simulink model "chap04_CA1"  (R2021a)
settings: Solver=FixedStepDiscrete  StartTime=0.0  StopTime=30  FixedStep=0.001  RelTol=1e-3
undefined symbols (not defined in the file): DiscIntNeverNeededParam
libraries: simulink x4
(part 3 of 4)

== system chap04_CA1/Subsystem/Subsystem2/Subsystem6 ==
  xx2 : Inport
  xx1 : Inport  Port=2
  xx4 : Inport  Port=3
  xx6 : Inport  Port=4
  vx2 : Inport  Port=5
  vx1 : Inport  Port=6
  vx4 : Inport  Port=7
  vx6 : Inport  Port=8
  Add : Sum
  Add{1,4,6,8} (4 alike) : Sum  Inputs=-+
  Add2 : Sum  Inputs=+-
  Add5 : Sum  Inputs=+++
  Add7 : Sum  Inputs=+-
  Add9 : Sum  Inputs=+++
  Constant1 : Constant  Value=0.5
  Constant2 : Constant  Value=1.0
  Constant3 : Constant  Value=0.5
  Constant4 : Constant  Value=1.0
  Constant5 : Constant  Value=1.5
  Constant6 : Constant  Value=1.5
  Gain : Gain  Gain=-5
  Product{3..5,7..9} (6 alike) : Product
  p2x : Outport
  wires:
  Product4/1 -> Add5/2
  Product5/1 -> Add5/3
  Constant3/1 -> Product4/1
  Add4/1 -> Product4/2
  xx2/1 -> Add1/2, Add4/2, Add2/1
  Constant4/1 -> Product5/2
  Add2/1 -> Product5/1
  xx4/1 -> Add4/1
  xx1/1 -> Add2/2
  xx6/1 -> Add1/1
  Constant5/1 -> Product3/1
  Add1/1 -> Product3/2
  Product3/1 -> Add5/1
  Product7/1 -> Add9/1
  Add6/1 -> Product7/2
  Constant6/1 -> Product7/1
  vx6/1 -> Add6/1
  vx1/1 -> Add7/2
  vx4/1 -> Add8/1
  Add7/1 -> Product9/1
  Constant2/1 -> Product9/2
  vx2/1 -> Add7/1, Add8/2, Add6/2
  Add8/1 -> Product8/2
  Constant1/1 -> Product8/1
  Product9/1 -> Add9/3
  Product8/1 -> Add9/2
  Add5/1 -> Add/1
  Add/1 -> Gain/1
  Gain/1 -> p2x/1
  Add9/1 -> Add/2

== system chap04_CA1/Subsystem/Subsystem3/Subsystem1 ==
  xy4 : Inport
  xy2 : Inport  Port=2
  xy3 : Inport  Port=3
  xy5 : Inport  Port=4
  vy4 : Inport  Port=5
  vy2 : Inport  Port=6
  vy3 : Inport  Port=7
  vy5 : Inport  Port=8
  Add : Sum
  Add{1,4,6,8} (4 alike) : Sum  Inputs=-+
  Add2 : Sum  Inputs=+-
  Add5 : Sum  Inputs=+++
  Add7 : Sum  Inputs=+-
  Add9 : Sum  Inputs=+++
  Constant3 : Constant  Value=1.0
  Constant4 : Constant  Value=0.5
  Constant5 : Constant  Value=1.2
  Constant6 : Constant  Value=1.0
  Constant7 : Constant  Value=0.5
  Constant8 : Constant  Value=1.2
  Gain : Gain  Gain=-5.0
  Product{3..5,7..9} (6 alike) : Product
  utx : Outport
  wires:
  Product4/1 -> Add5/2
  Product5/1 -> Add5/3
  Constant3/1 -> Product4/1
  Add4/1 -> Product4/2
  xy4/1 -> Add1/2, Add4/2, Add2/1
  Constant4/1 -> Product5/2
  Add2/1 -> Product5/1
  xy3/1 -> Add4/1
  xy2/1 -> Add2/2
  xy5/1 -> Add1/1
  Constant5/1 -> Product3/1
  Add1/1 -> Product3/2
  Product3/1 -> Add5/1
  Product7/1 -> Add9/1
  Add6/1 -> Product7/2
  Constant8/1 -> Product7/1
  vy5/1 -> Add6/1
  vy2/1 -> Add7/2
  vy3/1 -> Add8/1
  Add7/1 -> Product9/1
  Constant7/1 -> Product9/2
  vy4/1 -> Add7/1, Add8/2, Add6/2
  Add8/1 -> Product8/2
  Constant6/1 -> Product8/1
  Product9/1 -> Add9/3
  Product8/1 -> Add9/2
  Add5/1 -> Add/1
  Add/1 -> Gain/1
  Gain/1 -> utx/1
  Add9/1 -> Add/2

== system chap04_CA1/Subsystem/Subsystem3/Subsystem2 ==
  xz4 : Inport
  xx2 : Inport  Port=2
  xz3 : Inport  Port=3
  xz5 : Inport  Port=4
  vz4 : Inport  Port=5
  vz2 : Inport  Port=6
  vz3 : Inport  Port=7
  vz5 : Inport  Port=8
  Add : Sum
  Add{1,4,6,8} (4 alike) : Sum  Inputs=-+
  Add2 : Sum  Inputs=+-
  Add5 : Sum  Inputs=+++
  Add7 : Sum  Inputs=+-
  Add9 : Sum  Inputs=+++
  Constant3 : Constant  Value=1.0
  Constant4 : Constant  Value=0.5
  Constant5 : Constant  Value=1.2
  Constant6 : Constant  Value=1.0
  Constant7 : Constant  Value=0.5
  Constant8 : Constant  Value=1.2
  Gain : Gain  Gain=-5.0
  Product{3..5,7..9} (6 alike) : Product
  utx : Outport
  wires:
  Product8/1 -> Add9/2
  Product9/1 -> Add9/3
  Constant6/1 -> Product8/1
  Add8/1 -> Product8/2
  vz4/1 -> Add6/2, Add8/2, Add7/1
  Constant7/1 -> Product9/2
  Add7/1 -> Product9/1
  vz3/1 -> Add8/1
  vz2/1 -> Add7/2
  vz5/1 -> Add6/1
  Constant8/1 -> Product7/1
  Add6/1 -> Product7/2
  Product7/1 -> Add9/1
  Product3/1 -> Add5/1
  Add1/1 -> Product3/2
  Constant5/1 -> Product3/1
  xz5/1 -> Add1/1
  xx2/1 -> Add2/2
  xz3/1 -> Add4/1
  Add2/1 -> Product5/1
  Constant4/1 -> Product5/2
  xz4/1 -> Add2/1, Add4/2, Add1/2
  Add4/1 -> Product4/2
  Constant3/1 -> Product4/1
  Product5/1 -> Add5/3
  Product4/1 -> Add5/2
  Add5/1 -> Add/1
  Add/1 -> Gain/1
  Gain/1 -> utx/1
  Add9/1 -> Add/2

== system chap04_CA1/Subsystem/Subsystem3/Subsystem6 ==
  xx4 : Inport
  xx2 : Inport  Port=2
  xx3 : Inport  Port=3
  xx5 : Inport  Port=4
  vx4 : Inport  Port=5
  vx2 : Inport  Port=6
  vx3 : Inport  Port=7
  vx5 : Inport  Port=8
  Add : Sum
  Add{1,4,6,8} (4 alike) : Sum  Inputs=-+
  Add2 : Sum  Inputs=+-
  Add5 : Sum  Inputs=+++
  Add7 : Sum  Inputs=+-
  Add9 : Sum  Inputs=+++
  Constant3 : Constant  Value=1.0
  Constant4 : Constant  Value=0.5
  Constant5 : Constant  Value=1.2
  Constant6 : Constant  Value=1.0
  Constant7 : Constant  Value=0.5
  Constant8 : Constant  Value=1.2
  Gain : Gain  Gain=-5.0
  Product{3..5,7..9} (6 alike) : Product
  utx : Outport
  wires:
  Product8/1 -> Add9/2
  Product9/1 -> Add9/3
  Constant6/1 -> Product8/1
  Add8/1 -> Product8/2
  vx4/1 -> Add6/2, Add8/2, Add7/1
  Constant7/1 -> Product9/2
  Add7/1 -> Product9/1
  vx3/1 -> Add8/1
  vx2/1 -> Add7/2
  vx5/1 -> Add6/1
  Constant8/1 -> Product7/1
  Add6/1 -> Product7/2
  Product7/1 -> Add9/1
  Product3/1 -> Add5/1
  Add1/1 -> Product3/2
  Constant5/1 -> Product3/1
  xx5/1 -> Add1/1
  xx2/1 -> Add2/2
  xx3/1 -> Add4/1
  Add2/1 -> Product5/1
  Constant4/1 -> Product5/2
  xx4/1 -> Add2/1, Add4/2, Add1/2
  Add4/1 -> Product4/2
  Constant3/1 -> Product4/1
  Product5/1 -> Add5/3
  Product4/1 -> Add5/2
  Add5/1 -> Add/1
  Add/1 -> Gain/1
  Gain/1 -> utx/1
  Add9/1 -> Add/2

== system chap04_CA1/Subsystem/Subsystem4/Subsystem1 ==
  xx6 : Inport
  xx0 : Inport  Port=2
  xx1 : Inport  Port=3
  xx2 : Inport  Port=4
  vx6 : Inport  Port=5
  vx0 : Inport  Port=6
  vx1 : Inport  Port=7
  vx2 : Inport  Port=8
  Add : Sum
  Add1 : Sum  Inputs=-+
  Add10 : Sum  Inputs=-+
  Add2 : Sum  Inputs=+-
  Add4 : Sum  Inputs=-+
  Add5 : Sum  Inputs=+++
  Add6 : Sum  Inputs=+-
  Add8 : Sum  Inputs=+++
  Add9 : Sum  Inputs=+-
  Constant3 : Constant  Value=1.2
  Constant4 : Constant  Value=1.5
  Constant5 : Constant  Value=1.5
  Constant6 : Constant  Value=1.2
  Constant7 : Constant  Value=2.0
  Constant8 : Constant  Value=2.0
  Gain : Gain  Gain=-5.0
  Product{3..5,7..9} (6 alike) : Product
  utx : Outport
  wires:
  Product7/1 -> Add8/3
  Add6/1 -> Product7/1
  Constant8/1 -> Product7/2
  vx0/1 -> Add6/2
  Product3/1 -> Add5/1
  Add1/1 -> Product3/2
  Constant7/1 -> Product3/1
  xx0/1 -> Add1/1
  vx6/1 -> Add10/2, Add9/1, Add6/1
  vx2/1 -> Add10/1
  vx1/1 -> Add9/2
  xx1/1 -> Add2/2
  xx2/1 -> Add4/1
  Add2/1 -> Product5/1
  Constant3/1 -> Product5/2
  xx6/1 -> Add4/2, Add2/1, Add1/2
  Add4/1 -> Product4/2
  Constant4/1 -> Product4/1
  Product5/1 -> Add5/3
  Product4/1 -> Add5/2
  Constant5/1 -> Product8/1
  Add10/1 -> Product8/2
  Constant6/1 -> Product9/2
  Add9/1 -> Product9/1
  Product8/1 -> Add8/1
  Product9/1 -> Add8/2
  Add/1 -> Gain/1
  Gain/1 -> utx/1
  Add5/1 -> Add/1
  Add8/1 -> Add/2

== system chap04_CA1/Subsystem/Subsystem4/Subsystem2 ==
  xx6 : Inport
  xx0 : Inport  Port=2
  xx1 : Inport  Port=3
  xx2 : Inport  Port=4
  vx6 : Inport  Port=5
  vx0 : Inport  Port=6
  vx1 : Inport  Port=7
  vx2 : Inport  Port=8
  Add : Sum
  Add1 : Sum  Inputs=-+
  Add10 : Sum  Inputs=-+
  Add2 : Sum  Inputs=+-
  Add4 : Sum  Inputs=-+
  Add5 : Sum  Inputs=+++
  Add6 : Sum  Inputs=+-
  Add8 : Sum  Inputs=+++
  Add9 : Sum  Inputs=+-
  Constant3 : Constant  Value=1.2
  Constant4 : Constant  Value=1.5
  Constant5 : Constant  Value=1.5
  Constant6 : Constant  Value=1.2
  Constant7 : Constant  Value=2.0
  Constant8 : Constant  Value=2.0
  Gain : Gain  Gain=-5.0
  Product{3..5,7..9} (6 alike) : Product
  utx : Outport
  wires:
  Product9/1 -> Add8/2
  Product8/1 -> Add8/1
  Add9/1 -> Product9/1
  Constant6/1 -> Product9/2
  Add10/1 -> Product8/2
  Constant5/1 -> Product8/1
  Product4/1 -> Add5/2
  Product5/1 -> Add5/3
  Constant4/1 -> Product4/1
  Add4/1 -> Product4/2
  xx6/1 -> Add1/2, Add2/1, Add4/2
  Constant3/1 -> Product5/2
  Add2/1 -> Product5/1
  xx2/1 -> Add4/1
  xx1/1 -> Add2/2
  vx1/1 -> Add9/2
  vx2/1 -> Add10/1
  vx6/1 -> Add6/1, Add9/1, Add10/2
  xx0/1 -> Add1/1
  Constant7/1 -> Product3/1
  Add1/1 -> Product3/2
  Product3/1 -> Add5/1
  vx0/1 -> Add6/2
  Constant8/1 -> Product7/2
  Add6/1 -> Product7/1
  Product7/1 -> Add8/3
  Add/1 -> Gain/1
  Gain/1 -> utx/1
  Add5/1 -> Add/1
  Add8/1 -> Add/2

== system chap04_CA1/Subsystem/Subsystem4/Subsystem6 ==
  xx6 : Inport
  xx0 : Inport  Port=2
  xx1 : Inport  Port=3
  xx2 : Inport  Port=4
  vx6 : Inport  Port=5
  vx0 : Inport  Port=6
  vx1 : Inport  Port=7
  vx2 : Inport  Port=8
  Add : Sum
  Add1 : Sum  Inputs=-+
  Add10 : Sum  Inputs=-+
  Add2 : Sum  Inputs=+-
  Add4 : Sum  Inputs=-+
  Add5 : Sum  Inputs=+++
  Add6 : Sum  Inputs=+-
  Add8 : Sum  Inputs=+++
  Add9 : Sum  Inputs=+-
  Constant3 : Constant  Value=1.2
  Constant4 : Constant  Value=1.5
  Constant5 : Constant  Value=1.5
  Constant6 : Constant  Value=1.2
  Constant7 : Constant  Value=2.0
  Constant8 : Constant  Value=2.0
  Gain : Gain  Gain=-5.0
  Product{3..5,7..9} (6 alike) : Product
  utx : Outport
  wires:
  Product9/1 -> Add8/2
  Product8/1 -> Add8/1
  Add9/1 -> Product9/1
  Constant6/1 -> Product9/2
  Add10/1 -> Product8/2
  Constant5/1 -> Product8/1
  Product4/1 -> Add5/2
  Product5/1 -> Add5/3
  Constant4/1 -> Product4/1
  Add4/1 -> Product4/2
  xx6/1 -> Add1/2, Add2/1, Add4/2
  Constant3/1 -> Product5/2
  Add2/1 -> Product5/1
  xx2/1 -> Add4/1
  xx1/1 -> Add2/2
  vx1/1 -> Add9/2
  vx2/1 -> Add10/1
  vx6/1 -> Add6/1, Add9/1, Add10/2
  xx0/1 -> Add1/1
  Constant7/1 -> Product3/1
  Add1/1 -> Product3/2
  Product3/1 -> Add5/1
  vx0/1 -> Add6/2
  Constant8/1 -> Product7/2
  Add6/1 -> Product7/1
  Product7/1 -> Add8/3
  Add/1 -> Gain/1
  Gain/1 -> utx/1
  Add5/1 -> Add/1
  Add8/1 -> Add/2

== system chap04_CA1/Subsystem/Subsystem5/Subsystem1 ==
  xy3 : Inport
  xy1 : Inport  Port=2
  xy4 : Inport  Port=3
  xy5 : Inport  Port=4
  vy3 : Inport  Port=5
  vy1 : Inport  Port=6
  vy4 : Inport  Port=7
  vy5 : Inport  Port=8
  Add : Sum
  Add{1,4,6,8} (4 alike) : Sum  Inputs=-+
  Add2 : Sum  Inputs=+-
  Add5 : Sum  Inputs=+++
  Add7 : Sum  Inputs=+-
  Add9 : Sum  Inputs=+++
  Constant3 : Constant  Value=1.0
  Constant4 : Constant  Value=0.5
  Constant5 : Constant  Value=1.5
  Constant6 : Constant  Value=1.0
  Constant7 : Constant  Value=0.5
  Constant8 : Constant  Value=1.5
  Gain : Gain  Gain=-5
  Product{3..5,7..9} (6 alike) : Product
  p3y : Outport
  wires:
  Product4/1 -> Add5/2
  Product5/1 -> Add5/3
  Constant3/1 -> Product4/1
  Add4/1 -> Product4/2
  xy3/1 -> Add1/2, Add4/2, Add2/1
  Constant4/1 -> Product5/2
  Add2/1 -> Product5/1
  xy4/1 -> Add4/1
  xy1/1 -> Add2/2
  xy5/1 -> Add1/1
  Constant5/1 -> Product3/1
  Add1/1 -> Product3/2
  Product3/1 -> Add5/1
  Product7/1 -> Add9/1
  Add6/1 -> Product7/2
  Constant8/1 -> Product7/1
  vy5/1 -> Add6/1
  vy1/1 -> Add7/2
  vy4/1 -> Add8/1
  Add7/1 -> Product9/1
  Constant7/1 -> Product9/2
  vy3/1 -> Add7/1, Add8/2, Add6/2
  Add8/1 -> Product8/2
  Constant6/1 -> Product8/1
  Product9/1 -> Add9/3
  Product8/1 -> Add9/2
  Add/1 -> Gain/1
  Add5/1 -> Add/1
  Gain/1 -> p3y/1
  Add9/1 -> Add/2

== system chap04_CA1/Subsystem/Subsystem5/Subsystem2 ==
  xz3 : Inport
  xz1 : Inport  Port=2
  xz4 : Inport  Port=3
  xz5 : Inport  Port=4
  vz3 : Inport  Port=5
  vz1 : Inport  Port=6
  vz4 : Inport  Port=7
  vz5 : Inport  Port=8
  Add : Sum
  Add{1,4,6,8} (4 alike) : Sum  Inputs=-+
  Add2 : Sum  Inputs=+-
  Add5 : Sum  Inputs=+++
  Add7 : Sum  Inputs=+-
  Add9 : Sum  Inputs=+++
  Constant3 : Constant  Value=1.0
  Constant4 : Constant  Value=0.5
  Constant5 : Constant  Value=1.5
  Constant6 : Constant  Value=1.0
  Constant7 : Constant  Value=0.5
  Constant8 : Constant  Value=1.5
  Gain : Gain  Gain=-5
  Product{3..5,7..9} (6 alike) : Product
  p3z : Outport
  wires:
  Product8/1 -> Add9/2
  Product9/1 -> Add9/3
  Constant6/1 -> Product8/1
  Add8/1 -> Product8/2
  vz3/1 -> Add6/2, Add8/2, Add7/1
  Constant7/1 -> Product9/2
  Add7/1 -> Product9/1
  vz4/1 -> Add8/1
  vz1/1 -> Add7/2
  vz5/1 -> Add6/1
  Constant8/1 -> Product7/1
  Add6/1 -> Product7/2
  Product7/1 -> Add9/1
  Product3/1 -> Add5/1
  Add1/1 -> Product3/2
  Constant5/1 -> Product3/1
  xz5/1 -> Add1/1
  xz1/1 -> Add2/2
  xz4/1 -> Add4/1
  Add2/1 -> Product5/1
  Constant4/1 -> Product5/2
  xz3/1 -> Add2/1, Add4/2, Add1/2
  Add4/1 -> Product4/2
  Constant3/1 -> Product4/1
  Product5/1 -> Add5/3
  Product4/1 -> Add5/2
  Add5/1 -> Add/1
  Add/1 -> Gain/1
  Gain/1 -> p3z/1
  Add9/1 -> Add/2

== system chap04_CA1/Subsystem/Subsystem5/Subsystem6 ==
  xx3 : Inport
  xx1 : Inport  Port=2
  xx4 : Inport  Port=3
  xx5 : Inport  Port=4
  vx3 : Inport  Port=5
  vx1 : Inport  Port=6
  vx4 : Inport  Port=7
  vx5 : Inport  Port=8
  Add : Sum
  Add{1,4,6,8} (4 alike) : Sum  Inputs=-+
  Add2 : Sum  Inputs=+-
  Add5 : Sum  Inputs=+++
  Add7 : Sum  Inputs=+-
  Add9 : Sum  Inputs=+++
  Constant3 : Constant  Value=1.0
  Constant4 : Constant  Value=0.5
  Constant5 : Constant  Value=1.5
  Constant6 : Constant  Value=1.0
  Constant7 : Constant  Value=0.5
  Constant8 : Constant  Value=1.5
  Gain : Gain  Gain=-5
  Product{3..5,7..9} (6 alike) : Product
  p3x : Outport
  wires:
  Product8/1 -> Add9/2
  Product9/1 -> Add9/3
  Constant6/1 -> Product8/1
  Add8/1 -> Product8/2
  vx3/1 -> Add6/2, Add8/2, Add7/1
  Constant7/1 -> Product9/2
  Add7/1 -> Product9/1
  vx4/1 -> Add8/1
  vx1/1 -> Add7/2
  vx5/1 -> Add6/1
  Constant8/1 -> Product7/1
  Add6/1 -> Product7/2
  Product7/1 -> Add9/1
  Product3/1 -> Add5/1
  Add1/1 -> Product3/2
  Constant5/1 -> Product3/1
  xx5/1 -> Add1/1
  xx1/1 -> Add2/2
  xx4/1 -> Add4/1
  Add2/1 -> Product5/1
  Constant4/1 -> Product5/2
  xx3/1 -> Add2/1, Add4/2, Add1/2
  Add4/1 -> Product4/2
  Constant3/1 -> Product4/1
  Product5/1 -> Add5/3
  Product4/1 -> Add5/2
  Add5/1 -> Add/1
  Add/1 -> Gain/1
  Gain/1 -> p3x/1
  Add9/1 -> Add/2

== system chap04_CA1/Subsystem/Subsystem6/Subsystem ==
  In4 : Inport
  Add : Sum
  Bus Selector4 : BusSelector  OutputSignals=state(tk).node1.xx,state(t).node1.xx
  Bus Selector5 : BusSelector  OutputSignals=state(tk).node1.xy,state(t).node1.xy
  Bus Selector6 : BusSelector  OutputSignals=state(tk).node1.xz,state(t).node1.xz
  Bus Selector7 : BusSelector  OutputSignals=state(tk).node1.vx,state(t).node1.vx
  Bus Selector8 : BusSelector  OutputSignals=state(tk).node1.vy,state(t).node1.vy
  Bus Selector9 : BusSelector  OutputSignals=state(tk).node1.vz,state(t).node1.vz
  MATLAB Function1 : MATLAB Function  TreatAsAtomicUnit=on
  MATLAB Function2 : MATLAB Function  TreatAsAtomicUnit=on
  Mux1 : Mux  Inputs=3
  Mux2 : Mux  Inputs=3
  Square : Math  Operator=square  SaturateOnIntegerOverflow=on
  Square1 : Math  Operator=square  SaturateOnIntegerOverflow=on
  Subsystem3 : Subsystem
  Subsystem4 : Subsystem
  Subsystem5 : Subsystem
  Subsystem7 : Subsystem
  Subsystem8 : Subsystem
  Subsystem9 : Subsystem
  Out5 : Outport
  wires:
  Subsystem8/1(ez) -> Mux2/3
  Bus Selector4/1 -> Subsystem5/1(xxk)  "<xx>"
  Bus Selector4/2 -> Subsystem5/2(xx)  "<xx>"
  Subsystem7/1(ey) -> Mux2/2
  Bus Selector6/2 -> Subsystem4/2(xz)  "<xz>"
  Bus Selector5/2 -> Subsystem3/2(xy)  "<xy>"
  Subsystem5/1(exx) -> Mux1/1
  Subsystem9/1(evx) -> Mux2/1
  Subsystem3/1(exy) -> Mux1/2
  Subsystem4/1(exz) -> Mux1/3
  Mux1/1 -> MATLAB Function2/1(u)
  Bus Selector5/1 -> Subsystem3/1(xyk)  "<xy>"
  Bus Selector6/1 -> Subsystem4/1(xzk)  "<xz>"
  In4/1 -> Bus Selector9/1, Bus Selector8/1, Bus Selector7/1, Bus Selector6/1, Bus Selector5/1, Bus Selector4/1
  Add/1 -> Out5/1
  Bus Selector7/1 -> Subsystem9/1(vxk)  "<vx>"
  Bus Selector7/2 -> Subsystem9/2(vx)  "<vx>"
  Bus Selector8/1 -> Subsystem7/1(vyk)  "<vy>"
  Bus Selector8/2 -> Subsystem7/2(vy)  "<vy>"
  Bus Selector9/1 -> Subsystem8/1(vzk)  "<vz>"
  Bus Selector9/2 -> Subsystem8/2(vz)  "<vz>"
  Mux2/1 -> MATLAB Function1/1(u)
  MATLAB Function1/1(y) -> Square1/1
  MATLAB Function2/1(y) -> Square/1
  Square/1 -> Add/1
  Square1/1 -> Add/2

== system chap04_CA1/Subsystem/Subsystem6/Subsystem7 ==
  In1 : Inport
  Add : Sum  Inputs=+++
  Bus Selector : BusSelector  OutputSignals=state(tk).node1.xx,state(tk).node2.xx,state(tk).node3.xx,state(tk).node6.xx
  Bus Selector1 : BusSelector  OutputSignals=state(tk).node1.xy,state(tk).node2.xy,state(tk).node3.xy,state(tk).node6.xy
  Bus Selector2 : BusSelector  OutputSignals=state(tk).node1.xz,state(tk).node2.xz,state(tk).node3.xz,state(tk).node6.xz
  Bus Selector3 : BusSelector  OutputSignals=state(tk).node1.vx,state(tk).node2.vx,state(tk).node3.vx,state(tk).node6.vx
  Bus Selector4 : BusSelector  OutputSignals=state(tk).node1.vy,state(tk).node2.vy,state(tk).node3.vy,state(tk).node6.vy
  Bus Selector5 : BusSelector  OutputSignals=state(tk).node1.vz,state(tk).node2.vz,state(tk).node3.vz,state(tk).node6.vz
  Clock : Clock
  Constant : Constant  Value=-0.1
  Constant1 : Constant  Value=0.1
  Gain : Gain  Gain=0.1
  Gain1 : Gain  Gain=0.1
  MATLAB Function : MATLAB Function  TreatAsAtomicUnit=on
  MATLAB Function1 : MATLAB Function  TreatAsAtomicUnit=on
  Mux1 : Mux  Inputs=3
  Mux2 : Mux  Inputs=3
  Product : Product
  Product1 : Product
  Square : Math  Operator=square  SaturateOnIntegerOverflow=on
  Square1 : Math  Operator=square  SaturateOnIntegerOverflow=on
  Square2 : Math  SaturateOnIntegerOverflow=on
  Subsystem1 : Subsystem
  Subsystem2 : Subsystem
  Subsystem3 : Subsystem
  Subsystem4 : Subsystem
  Subsystem5 : Subsystem
  Subsystem6 : Subsystem
  Out1 : Outport
  wires:
  Bus Selector2/4 -> Subsystem2/4(xz6)  "<xz>"
  Bus Selector1/2 -> Subsystem1/2(xy2)  "<xy>"
  Subsystem2/1(pxz) -> Mux2/3
  Bus Selector2/1 -> Subsystem2/1(xz1)  "<xz>"
  Subsystem1/1(pxy) -> Mux2/2
  Bus Selector1/4 -> Subsystem1/4(xy6)  "<xy>"
  Bus Selector1/1 -> Subsystem1/1(xy1)  "<xy>"
  Mux2/1 -> MATLAB Function/1(u)
  Bus Selector2/3 -> Subsystem2/3(xz3)  "<xz>"
  Subsystem6/1(pxx) -> Mux2/1
  Bus Selector1/3 -> Subsystem1/3(xy3)  "<xy>"
  Bus Selector2/2 -> Subsystem2/2(xx2)  "<xz>"
  Add/1 -> Out1/1
  MATLAB Function/1(y) -> Square/1
  Bus Selector4/3 -> Subsystem3/3(vy3)  "<vy>"
  Subsystem5/1(pvx) -> Mux1/1
  Bus Selector3/2 -> Subsystem5/2(vx2)  "<vx>"
  Bus Selector4/2 -> Subsystem3/2(vy2)  "<vy>"
  Bus Selector5/2 -> Subsystem4/2(vz2)  "<vz>"
  Bus Selector3/1 -> Subsystem5/1(vx1)  "<vx>"
  Bus Selector3/3 -> Subsystem5/3(vx3)  "<vx>"
  Mux1/1 -> MATLAB Function1/1(u)
  Bus Selector4/1 -> Subsystem3/1(vy1)  "<vy>"
  Bus Selector5/4 -> Subsystem4/4(vz6)  "<vz>"
  Bus Selector4/4 -> Subsystem3/4(vy6)  "<vy>"
  In1/1 -> Bus Selector5/1, Bus Selector4/1, Bus Selector3/1, Bus Selector/1, Bus Selector1/1, Bus Selector2/1
  Bus Selector3/4 -> Subsystem5/4(vx6)  "<vx>"
  Bus Selector5/3 -> Subsystem4/3(vz3)  "<vz>"
  Bus Selector5/1 -> Subsystem4/1(vz1)  "<vz>"
  Subsystem3/1(pvy) -> Mux1/2
  Subsystem4/1(pvz) -> Mux1/3
  Bus Selector/1 -> Subsystem6/1(xx1)  "<xx>"
  Bus Selector/2 -> Subsystem6/2(xx2)  "<xx>"
  Bus Selector/3 -> Subsystem6/3(xx3)  "<xx>"
  Bus Selector/4 -> Subsystem6/4(xx6)  "<xx>"
  MATLAB Function1/1(y) -> Square1/1
  Product/1 -> Add/2
  Gain1/1 -> Add/1
  Gain/1 -> Add/3
  Square/1 -> Gain1/1
  Square1/1 -> Gain/1
  Square2/1 -> Product/1
  Clock/1 -> Product1/1
  Product1/1 -> Square2/1
  Constant/1 -> Product1/2
  Constant1/1 -> Product/2

== system chap04_CA1/Subsystem/Subsystem7/Subsystem7 ==
  In4 : Inport
  Add : Sum
  Bus Selector10 : BusSelector  OutputSignals=state(tk).node5.xx,state(t).node5.xx
  Bus Selector11 : BusSelector  OutputSignals=state(tk).node5.xy,state(t).node5.xy
  Bus Selector12 : BusSelector  OutputSignals=state(tk).node5.xz,state(t).node5.xz
  Bus Selector7 : BusSelector  OutputSignals=state(tk).node5.vx,state(t).node5.vx
  Bus Selector8 : BusSelector  OutputSignals=state(tk).node5.vy,state(t).node5.vy
  Bus Selector9 : BusSelector  OutputSignals=state(tk).node5.vz,state(t).node5.vz
  MATLAB Function1 : MATLAB Function  TreatAsAtomicUnit=on
  MATLAB Function2 : MATLAB Function  TreatAsAtomicUnit=on
  Mux1 : Mux  Inputs=3
  Mux2 : Mux  Inputs=3
  Square : Math  Operator=square  SaturateOnIntegerOverflow=on
  Square1 : Math  Operator=square  SaturateOnIntegerOverflow=on
  Subsystem3 : Subsystem
  Subsystem4 : Subsystem
  Subsystem5 : Subsystem
  Subsystem7 : Subsystem
  Subsystem8 : Subsystem
  Subsystem9 : Subsystem
  Out5 : Outport
  wires:
  Subsystem8/1(ez) -> Mux2/3
  Subsystem7/1(ey) -> Mux2/2
  Subsystem5/1(exx) -> Mux1/1
  Subsystem9/1(evx) -> Mux2/1
  Subsystem3/1(exy) -> Mux1/2
  Subsystem4/1(exz) -> Mux1/3
  Bus Selector10/1 -> Subsystem5/1(xxk)  "<xx>"
  Bus Selector12/1 -> Subsystem4/1(xzk)  "<xz>"
  Bus Selector11/2 -> Subsystem3/2(xy)  "<xy>"
  Bus Selector10/2 -> Subsystem5/2(xx)  "<xx>"
  Bus Selector11/1 -> Subsystem3/1(xyk)  "<xy>"
  Bus Selector12/2 -> Subsystem4/2(xz)  "<xz>"
  In4/1 -> Bus Selector12/1, Bus Selector11/1, Bus Selector10/1, Bus Selector7/1, Bus Selector9/1, Bus Selector8/1
  Bus Selector7/1 -> Subsystem9/1(vxk)  "<vx>"
  Bus Selector7/2 -> Subsystem9/2(vx)  "<vx>"
  Bus Selector8/1 -> Subsystem7/1(vyk)  "<vy>"
  Bus Selector8/2 -> Subsystem7/2(vy)  "<vy>"
  Bus Selector9/1 -> Subsystem8/1(vzk)  "<vz>"
  Bus Selector9/2 -> Subsystem8/2(vz)  "<vz>"
  MATLAB Function2/1(y) -> Square/1
  Mux2/1 -> MATLAB Function1/1(u)
  Square/1 -> Add/1
  Square1/1 -> Add/2
  Mux1/1 -> MATLAB Function2/1(u)
  MATLAB Function1/1(y) -> Square1/1
  Add/1 -> Out5/1

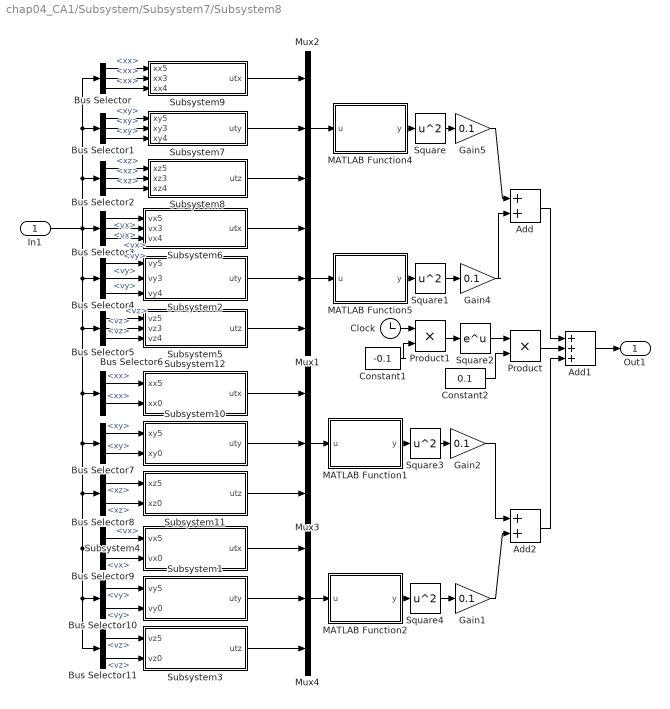
== system chap04_CA1/Subsystem/Subsystem7/Subsystem8 ==
  In1 : Inport
  Add : Sum
  Add1 : Sum  Inputs=+++
  Add2 : Sum
  Bus Selector : BusSelector  OutputSignals=state(tk).node5.xx,state(tk).node3.xx,state(tk).node4.xx
  Bus Selector1 : BusSelector  OutputSignals=state(tk).node5.xy,state(tk).node3.xy,state(tk).node4.xy
  Bus Selector10 : BusSelector  OutputSignals=state(t).node5.vy,state(t).node0.vy
  Bus Selector11 : BusSelector  OutputSignals=state(t).node5.vz,state(t).node0.vz
  Bus Selector2 : BusSelector  OutputSignals=state(tk).node5.xz,state(tk).node3.xz,state(tk).node4.xz
  Bus Selector3 : BusSelector  OutputSignals=state(tk).node5.vx,state(tk).node3.vx,state(tk).node4.vx
  Bus Selector4 : BusSelector  OutputSignals=state(tk).node5.vy,state(tk).node3.vy,state(tk).node4.vy
  Bus Selector5 : BusSelector  OutputSignals=state(tk).node5.vz,state(tk).node3.vz,state(tk).node4.vz
  Bus Selector6 : BusSelector  OutputSignals=state(t).node5.xx,state(t).node0.xx
  Bus Selector7 : BusSelector  OutputSignals=state(t).node5.xy,state(t).node0.xy
  Bus Selector8 : BusSelector  OutputSignals=state(t).node5.xz,state(t).node0.xz
  Bus Selector9 : BusSelector  OutputSignals=state(t).node5.vx,state(t).node0.vx
  Clock : Clock
  Constant1 : Constant  Value=-0.1
  Constant2 : Constant  Value=0.1
  Gain{1..2,4..5} (4 alike) : Gain  Gain=0.1
  MATLAB Function1 : MATLAB Function  TreatAsAtomicUnit=on
  MATLAB Function2 : MATLAB Function  TreatAsAtomicUnit=on
  MATLAB Function4 : MATLAB Function  TreatAsAtomicUnit=on
  MATLAB Function5 : MATLAB Function  TreatAsAtomicUnit=on
  Mux{1..4} (4 alike) : Mux  Inputs=3
  Product : Product
  Product1 : Product
  Square{,1,3..4} (4 alike) : Math  Operator=square  SaturateOnIntegerOverflow=on
  Square2 : Math  SaturateOnIntegerOverflow=on
  Subsystem1 : Subsystem
  Subsystem10 : Subsystem
  Subsystem11 : Subsystem
  Subsystem12 : Subsystem
  Subsystem2 : Subsystem
  Subsystem3 : Subsystem
  Subsystem4 : Subsystem
  Subsystem5 : Subsystem
  Subsystem6 : Subsystem
  Subsystem7 : Subsystem
  Subsystem8 : Subsystem
  Subsystem9 : Subsystem
  Out1 : Outport
  wires:
  Subsystem8/1(utz) -> Mux2/3
  Subsystem7/1(uty) -> Mux2/2
  Subsystem9/1(utx) -> Mux2/1
  Add/1 -> Add1/1
  Subsystem6/1(utx) -> Mux1/1
  In1/1 -> Bus Selector7/1, Bus Selector11/1, Bus Selector10/1, Bus Selector9/1, Bus Selector8/1, Bus Selector6/1, Bus Selector5/1, Bus Selector4/1, Bus Selector/1, Bus Selector1/1, Bus Selector2/1, Bus Selector3/1
  Subsystem2/1(uty) -> Mux1/2
  Subsystem5/1(utz) -> Mux1/3
  Bus Selector/1 -> Subsystem9/1(xx5)  "<xx>"
  Bus Selector/2 -> Subsystem9/2(xx3)  "<xx>"
  Bus Selector/3 -> Subsystem9/3(xx4)  "<xx>"
  Bus Selector1/1 -> Subsystem7/1(xy5)  "<xy>"
  Bus Selector1/2 -> Subsystem7/2(xy3)  "<xy>"
  Bus Selector1/3 -> Subsystem7/3(xy4)  "<xy>"
  Bus Selector2/1 -> Subsystem8/1(xz5)  "<xz>"
  Bus Selector2/2 -> Subsystem8/2(xz3)  "<xz>"
  Bus Selector2/3 -> Subsystem8/3(xz4)  "<xz>"
  Bus Selector4/2 -> Subsystem2/2(vy3)  "<vy>"
  Bus Selector4/1 -> Subsystem2/1(vy5)  "<vy>"
  Bus Selector4/3 -> Subsystem2/3(vy4)  "<vy>"
  Bus Selector3/1 -> Subsystem6/1(vx5)  "<vx>"
  Bus Selector3/2 -> Subsystem6/2(vx3)  "<vx>"
  Bus Selector3/3 -> Subsystem6/3(vx4)  "<vx>"
  Bus Selector5/3 -> Subsystem5/3(vz4)  "<vz>"
  Bus Selector5/2 -> Subsystem5/2(vz3)  "<vz>"
  Bus Selector5/1 -> Subsystem5/1(vz5)  "<vz>"
  Subsystem11/1(utz) -> Mux3/3
  Subsystem10/1(uty) -> Mux3/2
  Subsystem12/1(utx) -> Mux3/1
  Add1/1 -> Out1/1
  Add2/1 -> Add1/3
  Subsystem4/1(utx) -> Mux4/1
  Subsystem1/1(uty) -> Mux4/2
  Subsystem3/1(utz) -> Mux4/3
  Bus Selector6/2 -> Subsystem12/2(xx0)  "<xx>"
  Bus Selector6/1 -> Subsystem12/1(xx5)  "<xx>"
  Bus Selector7/1 -> Subsystem10/1(xy5)  "<xy>"
  Bus Selector7/2 -> Subsystem10/2(xy0)  "<xy>"
  Bus Selector8/1 -> Subsystem11/1(xz5)  "<xz>"
  Bus Selector8/2 -> Subsystem11/2(xz0)  "<xz>"
  Bus Selector9/1 -> Subsystem4/1(vx5)  "<vx>"
  Bus Selector9/2 -> Subsystem4/2(vx0)  "<vx>"
  Bus Selector10/1 -> Subsystem1/1(vy5)  "<vy>"
  Bus Selector10/2 -> Subsystem1/2(vy0)  "<vy>"
  Bus Selector11/1 -> Subsystem3/1(vz5)  "<vz>"
  Bus Selector11/2 -> Subsystem3/2(vz0)  "<vz>"
  Product/1 -> Add1/2
  MATLAB Function4/1(y) -> Square/1
  MATLAB Function5/1(y) -> Square1/1
  Square/1 -> Gain5/1
  Gain5/1 -> Add/1
  Square2/1 -> Product/1
  Constant1/1 -> Product1/2
  Product1/1 -> Square2/1
  Square1/1 -> Gain4/1
  Constant2/1 -> Product/2
  Clock/1 -> Product1/1
  Gain4/1 -> Add/2
  Mux2/1 -> MATLAB Function4/1(u)
  Mux1/1 -> MATLAB Function5/1(u)
  Mux4/1 -> MATLAB Function2/1(u)
  Mux3/1 -> MATLAB Function1/1(u)
  Gain1/1 -> Add2/2
  Square4/1 -> Gain1/1
  Gain2/1 -> Add2/1
  Square3/1 -> Gain2/1
  MATLAB Function2/1(y) -> Square4/1
  MATLAB Function1/1(y) -> Square3/1

== system chap04_CA1/Subsystem/Subsystem9/Subsystem7 ==
  In4 : Inport
  Add : Sum
  Bus Selector10 : BusSelector  OutputSignals=state(tk).node3.vx,state(t).node3.vx
  Bus Selector11 : BusSelector  OutputSignals=state(tk).node3.vy,state(t).node3.vy
  Bus Selector12 : BusSelector  OutputSignals=state(tk).node3.vz,state(t).node3.vz
  Bus Selector7 : BusSelector  OutputSignals=state(tk).node3.xx,state(t).node3.xx
  Bus Selector8 : BusSelector  OutputSignals=state(tk).node3.xy,state(t).node3.xy
  Bus Selector9 : BusSelector  OutputSignals=state(tk).node3.xz,state(t).node3.xz
  MATLAB Function1 : MATLAB Function  TreatAsAtomicUnit=on
  MATLAB Function2 : MATLAB Function  TreatAsAtomicUnit=on
  Mux1 : Mux  Inputs=3
  Mux2 : Mux  Inputs=3
  Square : Math  Operator=square  SaturateOnIntegerOverflow=on
  Square1 : Math  Operator=square  SaturateOnIntegerOverflow=on
  Subsystem3 : Subsystem
  Subsystem4 : Subsystem
  Subsystem5 : Subsystem
  Subsystem7 : Subsystem
  Subsystem8 : Subsystem
  Subsystem9 : Subsystem
  Out5 : Outport
  wires:
  Subsystem8/1(ez) -> Mux2/3
  Subsystem7/1(ey) -> Mux2/2
  Subsystem5/1(exx) -> Mux1/1
  Subsystem9/1(evx) -> Mux2/1
  Subsystem3/1(exy) -> Mux1/2
  Subsystem4/1(exz) -> Mux1/3
  Bus Selector7/1 -> Subsystem5/1(xxk)  "<xx>"
  Bus Selector9/1 -> Subsystem4/1(xzk)  "<xz>"
  Bus Selector8/2 -> Subsystem3/2(xy)  "<xy>"
  Bus Selector7/2 -> Subsystem5/2(xx)  "<xx>"
  Bus Selector8/1 -> Subsystem3/1(xyk)  "<xy>"
  Bus Selector9/2 -> Subsystem4/2(xz)  "<xz>"
  In4/1 -> Bus Selector9/1, Bus Selector8/1, Bus Selector7/1, Bus Selector10/1, Bus Selector12/1, Bus Selector11/1
  Bus Selector10/1 -> Subsystem9/1(vxk)  "<vx>"
  Bus Selector10/2 -> Subsystem9/2(vx)  "<vx>"
  Bus Selector11/1 -> Subsystem7/1(vyk)  "<vy>"
  Bus Selector11/2 -> Subsystem7/2(vy)  "<vy>"
  Bus Selector12/1 -> Subsystem8/1(vzk)  "<vz>"
  Bus Selector12/2 -> Subsystem8/2(vz)  "<vz>"
  MATLAB Function2/1(y) -> Square/1
  Mux2/1 -> MATLAB Function1/1(u)
  Square/1 -> Add/1
  Square1/1 -> Add/2
  Mux1/1 -> MATLAB Function2/1(u)
  MATLAB Function1/1(y) -> Square1/1
  Add/1 -> Out5/1

== system chap04_CA1/Subsystem/Subsystem9/Subsystem8 ==
  In1 : Inport
  Add : Sum  Inputs=+++
  Bus Selector : BusSelector  OutputSignals=state(tk).node3.xx,state(tk).node1.xx,state(tk).node4.xx,state(tk).node5.xx
  Bus Selector1 : BusSelector  OutputSignals=state(tk).node3.xy,state(tk).node1.xy,state(tk).node4.xy,state(tk).node5.xy
  Bus Selector2 : BusSelector  OutputSignals=state(tk).node3.xz,state(tk).node1.xz,state(tk).node4.xz,state(tk).node5.xz
  Bus Selector3 : BusSelector  OutputSignals=state(tk).node3.vx,state(tk).node1.vx,state(tk).node4.vx,state(tk).node5.vx
  Bus Selector4 : BusSelector  OutputSignals=state(tk).node3.vy,state(tk).node1.vy,state(tk).node4.vy,state(tk).node5.vy
  Bus Selector5 : BusSelector  OutputSignals=state(tk).node3.vz,state(tk).node1.vz,state(tk).node4.vz,state(tk).node5.vz
  Clock : Clock
  Constant : Constant  Value=-0.1
  Constant1 : Constant  Value=0.1
  Gain : Gain  Gain=0.1
  Gain1 : Gain  Gain=0.1
  MATLAB Function : MATLAB Function  TreatAsAtomicUnit=on
  MATLAB Function1 : MATLAB Function  TreatAsAtomicUnit=on
  Mux1 : Mux  Inputs=3
  Mux2 : Mux  Inputs=3
  Product : Product
  Product1 : Product
  Square : Math  Operator=square  SaturateOnIntegerOverflow=on
  Square1 : Math  Operator=square  SaturateOnIntegerOverflow=on
  Square2 : Math  SaturateOnIntegerOverflow=on
  Subsystem10 : Subsystem
  Subsystem11 : Subsystem
  Subsystem12 : Subsystem
  Subsystem7 : Subsystem
  Subsystem8 : Subsystem
  Subsystem9 : Subsystem
  Out1 : Outport
  wires:
  Bus Selector2/4 -> Subsystem11/4(xz5)  "<xz>"
  Bus Selector1/2 -> Subsystem10/2(xy1)  "<xy>"
  Subsystem11/1(p3z) -> Mux2/3
  Bus Selector2/1 -> Subsystem11/1(xz3)  "<xz>"
  Subsystem10/1(p3y) -> Mux2/2
  Bus Selector1/4 -> Subsystem10/4(xy5)  "<xy>"
  Bus Selector1/1 -> Subsystem10/1(xy3)  "<xy>"
  Bus Selector2/3 -> Subsystem11/3(xz4)  "<xz>"
  Subsystem12/1(p3x) -> Mux2/1
  Bus Selector1/3 -> Subsystem10/3(xy4)  "<xy>"
  Bus Selector2/2 -> Subsystem11/2(xz1)  "<xz>"
  Bus Selector4/3 -> Subsystem7/3(vy4)  "<vy>"
  Subsystem9/1(p3x) -> Mux1/1
  Bus Selector3/2 -> Subsystem9/2(vx1)  "<vx>"
  Bus Selector4/2 -> Subsystem7/2(vy1)  "<vy>"
  Bus Selector5/2 -> Subsystem8/2(vz1)  "<vz>"
  Bus Selector3/1 -> Subsystem9/1(vx3)  "<vx>"
  Bus Selector3/3 -> Subsystem9/3(vx4)  "<vx>"
  Bus Selector4/1 -> Subsystem7/1(vy3)  "<vy>"
  Bus Selector5/4 -> Subsystem8/4(vz5)  "<vz>"
  Bus Selector4/4 -> Subsystem7/4(vy5)  "<vy>"
  In1/1 -> Bus Selector3/1, Bus Selector5/1, Bus Selector4/1, Bus Selector2/1, Bus Selector1/1, Bus Selector/1
  Bus Selector3/4 -> Subsystem9/4(vx5)  "<vx>"
  Bus Selector5/3 -> Subsystem8/3(vz4)  "<vz>"
  Bus Selector5/1 -> Subsystem8/1(vz3)  "<vz>"
  Subsystem7/1(p3y) -> Mux1/2
  Subsystem8/1(p3z) -> Mux1/3
  Bus Selector/1 -> Subsystem12/1(xx3)  "<xx>"
  Bus Selector/2 -> Subsystem12/2(xx1)  "<xx>"
  Bus Selector/3 -> Subsystem12/3(xx4)  "<xx>"
  Bus Selector/4 -> Subsystem12/4(xx5)  "<xx>"
  Constant/1 -> Product1/2
  Square2/1 -> Product/1
  Constant1/1 -> Product/2
  Square1/1 -> Gain/1
  Gain/1 -> Add/3
  Product1/1 -> Square2/1
  Clock/1 -> Product1/1
  Add/1 -> Out1/1
  MATLAB Function/1(y) -> Square/1
  Mux1/1 -> MATLAB Function1/1(u)
  Square/1 -> Gain1/1
  MATLAB Function1/1(y) -> Square1/1
  Gain1/1 -> Add/1
  Mux2/1 -> MATLAB Function/1(u)
  Product/1 -> Add/2

== system chap04_CA1/Subsystem2/Subsystem7/Subsystem1 ==
  Abs1 : Abs
  Add : Sum  Inputs=+++
  Constant : Constant  Value=0.8
  Constant1 : Constant  Value=0.1
  Constant3 : Constant  Value=0.1
  Delay1 : Delay
  Delay2 : Delay  DelayLength=1
  Product{1..4} (4 alike) : Product
  Random Number1 : RandomNumber  Mean=0.75  Variance=0.5  Seed=2  SampleTime=0.01
  Repeating Sequence Interpolated2 : simulink/Sources/Repeating Sequence Interpolated  OutValues=[0.5 0.25 0.4 0.35 0.1].'  TimeValues=[0 0.1 0.5 0.6 1].'  LookUpMeth=Use Input Nearest  tsamp=1  OutMin=[]  OutMax=[]  OutDataTypeStr=double  OutputDataTypeScalingMode=double  OutDataType=fixdt(0,8)  OutScaling=2^-10
  Scope : Scope
  Out2 : Outport
  wires:
  Delay1/1 -> Product2/1
  Delay2/1 -> Product1/1
  Constant/1 -> Product2/2
  Constant3/1 -> Product1/2
  Constant1/1 -> Product3/2
  Product3/1 -> Add/1
  Product1/1 -> Add/2
  Product2/1 -> Add/3
  Product4/1 -> Product3/1
  Add/1 -> Out2/1, Delay1/1, Delay2/1
  Abs1/1 -> Product4/1, Scope/1
  Random Number1/1 -> Abs1/1
  Repeating Sequence Interpolated2/1 -> Product4/2

== system chap04_CA1/Subsystem2/Subsystem7/Subsystem2 ==
  In2 : Inport
  Add : Sum  Inputs=+++
  Constant : Constant  Value=0.8
  Constant1 : Constant  Value=0.1
  Constant3 : Constant  Value=0.1
  Delay1 : Delay
  Delay2 : Delay  DelayLength=1
  Product1 : Product
  Product2 : Product
  Product3 : Product
  Out2 : Outport
  wires:
  Add/1 -> Delay2/1, Delay1/1, Out2/1
  In2/1 -> Product3/1
  Product2/1 -> Add/3
  Product1/1 -> Add/2
  Product3/1 -> Add/1
  Constant1/1 -> Product3/2
  Constant3/1 -> Product1/2
  Constant/1 -> Product2/2
  Delay2/1 -> Product1/1
  Delay1/1 -> Product2/1

== system chap04_CA1/Subsystem2/Subsystem7/Subsystem3 ==
  In2 : Inport
  Add : Sum  Inputs=+++
  Constant : Constant  Value=0.8
  Constant1 : Constant  Value=0.1
  Constant3 : Constant  Value=0.1
  Delay1 : Delay
  Delay2 : Delay  DelayLength=1
  Product1 : Product
  Product2 : Product
  Product3 : Product
  Out2 : Outport
  wires:
  Delay1/1 -> Product2/1
  Delay2/1 -> Product1/1
  Constant/1 -> Product2/2
  Constant3/1 -> Product1/2
  Constant1/1 -> Product3/2
  Product3/1 -> Add/1
  Product1/1 -> Add/2
  Product2/1 -> Add/3
  In2/1 -> Product3/1
  Add/1 -> Out2/1, Delay1/1, Delay2/1

== system chap04_CA1/Subsystem2/Subsystem7/Subsystem4 ==
  In2 : Inport
  Add : Sum  Inputs=+++
  Constant : Constant  Value=0.8
  Constant1 : Constant  Value=0.1
  Constant3 : Constant  Value=0.1
  Delay1 : Delay
  Delay2 : Delay  DelayLength=1
  Product1 : Product
  Product2 : Product
  Product3 : Product
  Out2 : Outport
  wires:
  Add/1 -> Delay2/1, Delay1/1, Out2/1
  In2/1 -> Product3/1
  Product2/1 -> Add/3
  Product1/1 -> Add/2
  Product3/1 -> Add/1
  Constant1/1 -> Product3/2
  Constant3/1 -> Product1/2
  Constant/1 -> Product2/2
  Delay2/1 -> Product1/1
  Delay1/1 -> Product2/1

== system chap04_CA1/Subsystem/Subsystem10/Subsystem7/Subsystem3 ==
  xyk : Inport
  xy : Inport  Port=2
  Add4 : Sum  Inputs=-+
  exy : Outport
  wires:
  xy/1 -> Add4/1
  Add4/1 -> exy/1
  xyk/1 -> Add4/2

== system chap04_CA1/Subsystem/Subsystem10/Subsystem7/Subsystem4 ==
  xzk : Inport
  xz : Inport  Port=2
  Add4 : Sum  Inputs=-+
  exz : Outport
  wires:
  xzk/1 -> Add4/2
  Add4/1 -> exz/1
  xz/1 -> Add4/1

== system chap04_CA1/Subsystem/Subsystem10/Subsystem7/Subsystem5 ==
  xxk : Inport
  xx : Inport  Port=2
  Add4 : Sum  Inputs=-+
  exx : Outport
  wires:
  xxk/1 -> Add4/2
  Add4/1 -> exx/1
  xx/1 -> Add4/1

== system chap04_CA1/Subsystem/Subsystem10/Subsystem7/Subsystem7 ==
  vyk : Inport
  vy : Inport  Port=2
  Add8 : Sum  Inputs=-+
  ey : Outport
  wires:
  Add8/1 -> ey/1
  vy/1 -> Add8/1
  vyk/1 -> Add8/2

== system chap04_CA1/Subsystem/Subsystem10/Subsystem7/Subsystem8 ==
  vzk : Inport
  vz : Inport  Port=2
  Add8 : Sum  Inputs=-+
  ez : Outport
  wires:
  vzk/1 -> Add8/2
  vz/1 -> Add8/1
  Add8/1 -> ez/1

== system chap04_CA1/Subsystem/Subsystem10/Subsystem7/Subsystem9 ==
  vxk : Inport
  vx : Inport  Port=2
  Add8 : Sum  Inputs=-+
  evx : Outport
  wires:
  vxk/1 -> Add8/2
  vx/1 -> Add8/1
  Add8/1 -> evx/1

== system chap04_CA1/Subsystem/Subsystem10/Subsystem8/Subsystem10 ==
  xy4 : Inport
  xy2 : Inport  Port=2
  xy3 : Inport  Port=3
  xy5 : Inport  Port=4
  Add1 : Sum  Inputs=-+
  Add2 : Sum  Inputs=+-
  Add4 : Sum  Inputs=-+
  Add5 : Sum  Inputs=+++
  Constant3 : Constant  Value=1.0
  Constant4 : Constant  Value=0.5
  Constant5 : Constant  Value=1.2
  Product3 : Product
  Product4 : Product
  Product5 : Product
  p4y : Outport
  wires:
  Product3/1 -> Add5/1
  Add1/1 -> Product3/2
  Constant5/1 -> Product3/1
  xy5/1 -> Add1/1
  xy2/1 -> Add2/2
  xy3/1 -> Add4/1
  Add2/1 -> Product5/1
  Constant4/1 -> Product5/2
  xy4/1 -> Add2/1, Add4/2, Add1/2
  Add4/1 -> Product4/2
  Constant3/1 -> Product4/1
  Product5/1 -> Add5/3
  Product4/1 -> Add5/2
  Add5/1 -> p4y/1

== system chap04_CA1/Subsystem/Subsystem10/Subsystem8/Subsystem11 ==
  xz4 : Inport
  xx2 : Inport  Port=2
  xz3 : Inport  Port=3
  xz5 : Inport  Port=4
  Add1 : Sum  Inputs=-+
  Add2 : Sum  Inputs=+-
  Add4 : Sum  Inputs=-+
  Add5 : Sum  Inputs=+++
  Constant3 : Constant  Value=1.0
  Constant4 : Constant  Value=0.5
  Constant5 : Constant  Value=1.2
  Product3 : Product
  Product4 : Product
  Product5 : Product
  p4z : Outport
  wires:
  Product4/1 -> Add5/2
  Product5/1 -> Add5/3
  Constant3/1 -> Product4/1
  Add4/1 -> Product4/2
  xz4/1 -> Add1/2, Add4/2, Add2/1
  Constant4/1 -> Product5/2
  Add2/1 -> Product5/1
  xz3/1 -> Add4/1
  xx2/1 -> Add2/2
  xz5/1 -> Add1/1
  Constant5/1 -> Product3/1
  Add1/1 -> Product3/2
  Product3/1 -> Add5/1
  Add5/1 -> p4z/1

== system chap04_CA1/Subsystem/Subsystem10/Subsystem8/Subsystem12 ==
  xx4 : Inport
  xx2 : Inport  Port=2
  xx3 : Inport  Port=3
  xx5 : Inport  Port=4
  Add1 : Sum  Inputs=-+
  Add2 : Sum  Inputs=+-
  Add4 : Sum  Inputs=-+
  Add5 : Sum  Inputs=+++
  Constant3 : Constant  Value=1.0
  Constant4 : Constant  Value=0.5
  Constant5 : Constant  Value=1.2
  Product3 : Product
  Product4 : Product
  Product5 : Product
  p4x : Outport
  wires:
  Product4/1 -> Add5/2
  Product5/1 -> Add5/3
  Constant3/1 -> Product4/1
  Add4/1 -> Product4/2
  xx4/1 -> Add1/2, Add4/2, Add2/1
  Constant4/1 -> Product5/2
  Add2/1 -> Product5/1
  xx3/1 -> Add4/1
  xx2/1 -> Add2/2
  xx5/1 -> Add1/1
  Constant5/1 -> Product3/1
  Add1/1 -> Product3/2
  Product3/1 -> Add5/1
  Add5/1 -> p4x/1

== system chap04_CA1/Subsystem/Subsystem10/Subsystem8/Subsystem7 ==
  vy4 : Inport
  vy2 : Inport  Port=2
  vy3 : Inport  Port=3
  vy5 : Inport  Port=4
  Add6 : Sum  Inputs=-+
  Add7 : Sum  Inputs=+-
  Add8 : Sum  Inputs=-+
  Add9 : Sum  Inputs=+++
  Constant3 : Constant  Value=1.0
  Constant4 : Constant  Value=0.5
  Constant5 : Constant  Value=1.2
  Product7 : Product
  Product8 : Product
  Product9 : Product
  p4y : Outport
  wires:
  Product8/1 -> Add9/2
  Product9/1 -> Add9/3
  Constant3/1 -> Product8/1
  Add8/1 -> Product8/2
  vy4/1 -> Add6/2, Add8/2, Add7/1
  Constant4/1 -> Product9/2
  Add7/1 -> Product9/1
  vy3/1 -> Add8/1
  vy2/1 -> Add7/2
  vy5/1 -> Add6/1
  Constant5/1 -> Product7/1
  Add6/1 -> Product7/2
  Product7/1 -> Add9/1
  Add9/1 -> p4y/1

== system chap04_CA1/Subsystem/Subsystem10/Subsystem8/Subsystem8 ==
  vz4 : Inport
  vz2 : Inport  Port=2
  vz3 : Inport  Port=3
  vz5 : Inport  Port=4
  Add6 : Sum  Inputs=-+
  Add7 : Sum  Inputs=+-
  Add8 : Sum  Inputs=-+
  Add9 : Sum  Inputs=+++
  Constant3 : Constant  Value=1.0
  Constant4 : Constant  Value=0.5
  Constant5 : Constant  Value=1.2
  Product7 : Product
  Product8 : Product
  Product9 : Product
  p4z : Outport
  wires:
  Add9/1 -> p4z/1
  Product7/1 -> Add9/1
  Add6/1 -> Product7/2
  Constant5/1 -> Product7/1
  vz5/1 -> Add6/1
  vz2/1 -> Add7/2
  vz3/1 -> Add8/1
  Add7/1 -> Product9/1
  Constant4/1 -> Product9/2
  vz4/1 -> Add7/1, Add8/2, Add6/2
  Add8/1 -> Product8/2
  Constant3/1 -> Product8/1
  Product9/1 -> Add9/3
  Product8/1 -> Add9/2

== system chap04_CA1/Subsystem/Subsystem10/Subsystem8/Subsystem9 ==
  vx4 : Inport
  vx2 : Inport  Port=2
  vx3 : Inport  Port=3
  vx5 : Inport  Port=4
  Add6 : Sum  Inputs=-+
  Add7 : Sum  Inputs=+-
  Add8 : Sum  Inputs=-+
  Add9 : Sum  Inputs=+++
  Constant3 : Constant  Value=1.0
  Constant4 : Constant  Value=0.5
  Constant5 : Constant  Value=1.2
  Product7 : Product
  Product8 : Product
  Product9 : Product
  p4x : Outport
  wires:
  Product7/1 -> Add9/1
  Add6/1 -> Product7/2
  Constant5/1 -> Product7/1
  vx5/1 -> Add6/1
  vx2/1 -> Add7/2
  vx3/1 -> Add8/1
  Add7/1 -> Product9/1
  Constant4/1 -> Product9/2
  vx4/1 -> Add7/1, Add8/2, Add6/2
  Add8/1 -> Product8/2
  Constant3/1 -> Product8/1
  Product9/1 -> Add9/3
  Product8/1 -> Add9/2
  Add9/1 -> p4x/1

== system chap04_CA1/Subsystem/Subsystem11/Subsystem7/Subsystem3 ==
  xyk : Inport
  xy : Inport  Port=2
  Add4 : Sum  Inputs=-+
  exy : Outport
  wires:
  xy/1 -> Add4/1
  Add4/1 -> exy/1
  xyk/1 -> Add4/2

== system chap04_CA1/Subsystem/Subsystem11/Subsystem7/Subsystem4 ==
  xzk : Inport
  xz : Inport  Port=2
  Add4 : Sum  Inputs=-+
  exz : Outport
  wires:
  xzk/1 -> Add4/2
  Add4/1 -> exz/1
  xz/1 -> Add4/1

== system chap04_CA1/Subsystem/Subsystem11/Subsystem7/Subsystem5 ==
  xxk : Inport
  xx : Inport  Port=2
  Add4 : Sum  Inputs=-+
  exx : Outport
  wires:
  xxk/1 -> Add4/2
  Add4/1 -> exx/1
  xx/1 -> Add4/1

== system chap04_CA1/Subsystem/Subsystem11/Subsystem7/Subsystem7 ==
  vyk : Inport
  vy : Inport  Port=2
  Add8 : Sum  Inputs=-+
  ey : Outport
  wires:
  Add8/1 -> ey/1
  vy/1 -> Add8/1
  vyk/1 -> Add8/2

== system chap04_CA1/Subsystem/Subsystem11/Subsystem7/Subsystem8 ==
  vzk : Inport
  vz : Inport  Port=2
  Add8 : Sum  Inputs=-+
  ez : Outport
  wires:
  vzk/1 -> Add8/2
  vz/1 -> Add8/1
  Add8/1 -> ez/1

== system chap04_CA1/Subsystem/Subsystem11/Subsystem7/Subsystem9 ==
  vxk : Inport
  vx : Inport  Port=2
  Add8 : Sum  Inputs=-+
  evx : Outport
  wires:
  vxk/1 -> Add8/2
  vx/1 -> Add8/1
  Add8/1 -> evx/1

== system chap04_CA1/Subsystem/Subsystem11/Subsystem8/Subsystem13 ==
  xx6 : Inport
  xx0 : Inport  Port=2
  Add1 : Sum  Inputs=-+
  Constant7 : Constant  Value=2.0
  Product3 : Product
  utx : Outport
  wires:
  Add1/1 -> Product3/2
  Constant7/1 -> Product3/1
  xx0/1 -> Add1/1
  xx6/1 -> Add1/2
  Product3/1 -> utx/1

== system chap04_CA1/Subsystem/Subsystem11/Subsystem8/Subsystem14 ==
  xx6 : Inport
  xx0 : Inport  Port=2
  Add1 : Sum  Inputs=-+
  Constant7 : Constant  Value=2.0
  Product3 : Product
  utx : Outport
  wires:
  xx6/1 -> Add1/2
  xx0/1 -> Add1/1
  Constant7/1 -> Product3/1
  Add1/1 -> Product3/2
  Product3/1 -> utx/1

== system chap04_CA1/Subsystem/Subsystem11/Subsystem8/Subsystem15 ==
  xx6 : Inport
  xx0 : Inport  Port=2
  Add1 : Sum  Inputs=-+
  Constant7 : Constant  Value=2.0
  Product3 : Product
  utx : Outport
  wires:
  xx6/1 -> Add1/2
  xx0/1 -> Add1/1
  Constant7/1 -> Product3/1
  Add1/1 -> Product3/2
  Product3/1 -> utx/1

== system chap04_CA1/Subsystem/Subsystem11/Subsystem8/Subsystem16 ==
  vx6 : Inport
  vx1 : Inport  Port=2
  vx2 : Inport  Port=3
  Add10 : Sum  Inputs=-+
  Add8 : Sum
  Add9 : Sum  Inputs=+-
  Constant3 : Constant  Value=1.2
  Constant4 : Constant  Value=1.5
  Product8 : Product
  Product9 : Product
  utx : Outport
  wires:
  vx6/1 -> Add10/2, Add9/1
  vx2/1 -> Add10/1
  vx1/1 -> Add9/2
  Constant4/1 -> Product8/1
  Add10/1 -> Product8/2
  Constant3/1 -> Product9/2
  Add9/1 -> Product9/1
  Product8/1 -> Add8/1
  Product9/1 -> Add8/2
  Add8/1 -> utx/1

== system chap04_CA1/Subsystem/Subsystem11/Subsystem8/Subsystem17 ==
  vx6 : Inport
  vx1 : Inport  Port=2
  vx2 : Inport  Port=3
  Add10 : Sum  Inputs=-+
  Add8 : Sum
  Add9 : Sum  Inputs=+-
  Constant3 : Constant  Value=1.2
  Constant4 : Constant  Value=1.5
  Product8 : Product
  Product9 : Product
  utx : Outport
  wires:
  Product9/1 -> Add8/2
  Product8/1 -> Add8/1
  Add9/1 -> Product9/1
  Constant3/1 -> Product9/2
  Add10/1 -> Product8/2
  Constant4/1 -> Product8/1
  vx1/1 -> Add9/2
  vx2/1 -> Add10/1
  vx6/1 -> Add9/1, Add10/2
  Add8/1 -> utx/1

== system chap04_CA1/Subsystem/Subsystem11/Subsystem8/Subsystem18 ==
  vx6 : Inport
  vx1 : Inport  Port=2
  vx2 : Inport  Port=3
  Add10 : Sum  Inputs=-+
  Add8 : Sum
  Add9 : Sum  Inputs=+-
  Constant3 : Constant  Value=1.2
  Constant4 : Constant  Value=1.5
  Product8 : Product
  Product9 : Product
  utx : Outport
  wires:
  Product9/1 -> Add8/2
  Product8/1 -> Add8/1
  Add9/1 -> Product9/1
  Constant3/1 -> Product9/2
  Add10/1 -> Product8/2
  Constant4/1 -> Product8/1
  vx1/1 -> Add9/2
  vx2/1 -> Add10/1
  vx6/1 -> Add9/1, Add10/2
  Add8/1 -> utx/1

== system chap04_CA1/Subsystem/Subsystem11/Subsystem8/Subsystem19 ==
  xx6 : Inport
  xx1 : Inport  Port=2
  xx2 : Inport  Port=3
  Add2 : Sum  Inputs=+-
  Add4 : Sum  Inputs=-+
  Add5 : Sum
  Constant3 : Constant  Value=1.2
  Constant4 : Constant  Value=1.5
  Product4 : Product
  Product5 : Product
  utx : Outport
  wires:
  xx1/1 -> Add2/2
  xx2/1 -> Add4/1
  Add2/1 -> Product5/1
  Constant3/1 -> Product5/2
  xx6/1 -> Add4/2, Add2/1
  Add4/1 -> Product4/2
  Constant4/1 -> Product4/1
  Product5/1 -> Add5/2
  Product4/1 -> Add5/1
  Add5/1 -> utx/1

== system chap04_CA1/Subsystem/Subsystem11/Subsystem8/Subsystem2 ==
  vx6 : Inport
  vx0 : Inport  Port=2
  Add6 : Sum  Inputs=+-
  Constant8 : Constant  Value=2.0
  Product7 : Product
  utx : Outport
  wires:
  vx6/1 -> Add6/1
  vx0/1 -> Add6/2
  Constant8/1 -> Product7/2
  Add6/1 -> Product7/1
  Product7/1 -> utx/1

== system chap04_CA1/Subsystem/Subsystem11/Subsystem8/Subsystem20 ==
  xx6 : Inport
  xx1 : Inport  Port=2
  xx2 : Inport  Port=3
  Add2 : Sum  Inputs=+-
  Add4 : Sum  Inputs=-+
  Add5 : Sum
  Constant3 : Constant  Value=1.2
  Constant4 : Constant  Value=1.5
  Product4 : Product
  Product5 : Product
  utx : Outport
  wires:
  Product4/1 -> Add5/1
  Product5/1 -> Add5/2
  Constant4/1 -> Product4/1
  Add4/1 -> Product4/2
  xx6/1 -> Add2/1, Add4/2
  Constant3/1 -> Product5/2
  Add2/1 -> Product5/1
  xx2/1 -> Add4/1
  xx1/1 -> Add2/2
  Add5/1 -> utx/1

== system chap04_CA1/Subsystem/Subsystem11/Subsystem8/Subsystem21 ==
  xx6 : Inport
  xx1 : Inport  Port=2
  xx2 : Inport  Port=3
  Add2 : Sum  Inputs=+-
  Add4 : Sum  Inputs=-+
  Add5 : Sum
  Constant3 : Constant  Value=1.2
  Constant4 : Constant  Value=1.5
  Product4 : Product
  Product5 : Product
  utx : Outport
  wires:
  Product4/1 -> Add5/1
  Product5/1 -> Add5/2
  Constant4/1 -> Product4/1
  Add4/1 -> Product4/2
  xx6/1 -> Add2/1, Add4/2
  Constant3/1 -> Product5/2
  Add2/1 -> Product5/1
  xx2/1 -> Add4/1
  xx1/1 -> Add2/2
  Add5/1 -> utx/1

== system chap04_CA1/Subsystem/Subsystem11/Subsystem8/Subsystem5 ==
  vx6 : Inport
  vx0 : Inport  Port=2
  Add6 : Sum  Inputs=+-
  Constant8 : Constant  Value=2.0
  Product7 : Product
  utx : Outport
  wires:
  Add6/1 -> Product7/1
  Constant8/1 -> Product7/2
  vx0/1 -> Add6/2
  vx6/1 -> Add6/1
  Product7/1 -> utx/1

== system chap04_CA1/Subsystem/Subsystem11/Subsystem8/Subsystem6 ==
  vx6 : Inport
  vx0 : Inport  Port=2
  Add6 : Sum  Inputs=+-
  Constant8 : Constant  Value=2.0
  Product7 : Product
  utx : Outport
  wires:
  Add6/1 -> Product7/1
  Constant8/1 -> Product7/2
  vx0/1 -> Add6/2
  vx6/1 -> Add6/1
  Product7/1 -> utx/1

== system chap04_CA1/Subsystem/Subsystem13/Subsystem3/Subsystem3 ==
  xyk : Inport
  xy : Inport  Port=2
  Add4 : Sum  Inputs=-+
  exy : Outport
  wires:
  xy/1 -> Add4/1
  Add4/1 -> exy/1
  xyk/1 -> Add4/2

== system chap04_CA1/Subsystem/Subsystem13/Subsystem3/Subsystem4 ==
  xzk : Inport
  xz : Inport  Port=2
  Add4 : Sum  Inputs=-+
  exz : Outport
  wires:
  xzk/1 -> Add4/2
  Add4/1 -> exz/1
  xz/1 -> Add4/1

== system chap04_CA1/Subsystem/Subsystem13/Subsystem3/Subsystem5 ==
  xxk : Inport
  xx : Inport  Port=2
  Add4 : Sum  Inputs=-+
  exx : Outport
  wires:
  xxk/1 -> Add4/2
  Add4/1 -> exx/1
  xx/1 -> Add4/1

== system chap04_CA1/Subsystem/Subsystem13/Subsystem3/Subsystem7 ==
  vyk : Inport
  vy : Inport  Port=2
  Add8 : Sum  Inputs=-+
  ey : Outport
  wires:
  Add8/1 -> ey/1
  vy/1 -> Add8/1
  vyk/1 -> Add8/2

== system chap04_CA1/Subsystem/Subsystem13/Subsystem3/Subsystem8 ==
  vzk : Inport
  vz : Inport  Port=2
  Add8 : Sum  Inputs=-+
  ez : Outport
  wires:
  vzk/1 -> Add8/2
  vz/1 -> Add8/1
  Add8/1 -> ez/1

== system chap04_CA1/Subsystem/Subsystem13/Subsystem3/Subsystem9 ==
  vxk : Inport
  vx : Inport  Port=2
  Add8 : Sum  Inputs=-+
  evx : Outport
  wires:
  vxk/1 -> Add8/2
  vx/1 -> Add8/1
  Add8/1 -> evx/1

== system chap04_CA1/Subsystem/Subsystem13/Subsystem7/Subsystem10 ==
  xy2 : Inport
  xy1 : Inport  Port=2
  xy4 : Inport  Port=3
  xy6 : Inport  Port=4
  Add1 : Sum  Inputs=-+
  Add2 : Sum  Inputs=+-
  Add4 : Sum  Inputs=-+
  Add5 : Sum  Inputs=+++
  Constant3 : Constant  Value=0.5
  Constant4 : Constant  Value=1.0
  Constant5 : Constant  Value=1.5
  Product3 : Product
  Product4 : Product
  Product5 : Product
  p2y : Outport
  wires:
  Product3/1 -> Add5/1
  Add1/1 -> Product3/2
  Constant5/1 -> Product3/1
  xy6/1 -> Add1/1
  xy1/1 -> Add2/2
  xy4/1 -> Add4/1
  Add2/1 -> Product5/1
  Constant4/1 -> Product5/2
  xy2/1 -> Add2/1, Add4/2, Add1/2
  Add4/1 -> Product4/2
  Constant3/1 -> Product4/1
  Product5/1 -> Add5/3
  Product4/1 -> Add5/2
  Add5/1 -> p2y/1

== system chap04_CA1/Subsystem/Subsystem13/Subsystem7/Subsystem11 ==
  xz2 : Inport
  xz1 : Inport  Port=2
  xz4 : Inport  Port=3
  xz6 : Inport  Port=4
  Add1 : Sum  Inputs=-+
  Add2 : Sum  Inputs=+-
  Add4 : Sum  Inputs=-+
  Add5 : Sum  Inputs=+++
  Constant3 : Constant  Value=0.5
  Constant4 : Constant  Value=1.0
  Constant5 : Constant  Value=1.5
  Product3 : Product
  Product4 : Product
  Product5 : Product
  p2z : Outport
  wires:
  Product4/1 -> Add5/2
  Product5/1 -> Add5/3
  Constant3/1 -> Product4/1
  Add4/1 -> Product4/2
  xz2/1 -> Add1/2, Add4/2, Add2/1
  Constant4/1 -> Product5/2
  Add2/1 -> Product5/1
  xz4/1 -> Add4/1
  xz1/1 -> Add2/2
  xz6/1 -> Add1/1
  Constant5/1 -> Product3/1
  Add1/1 -> Product3/2
  Product3/1 -> Add5/1
  Add5/1 -> p2z/1
